simulink model "simulaciones_controlador"  (R2021a)
settings: Solver=VariableStepAuto  StartTime=0.0  StopTime=10.0  RelTol=1e-3
libraries: cstblocks x2
settings Model: Creator=camid  LastModifiedBy=camid

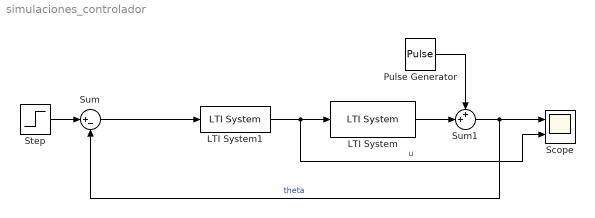
== system simulaciones_controlador ==
  LTI System : cstblocks/LTI System  sys=Planta  IC=[]
  LTI System1 : cstblocks/LTI System  sys=C  IC=[]
  Pulse Generator : DiscretePulseGenerator  PulseType=Time based  Amplitude=10  Period=30  PulseWidth=0.1  PhaseDelay=2
  Scope : Scope  NumInputPorts=2
  Step : Step  After=0  SampleTime=0
  Sum : Sum  Inputs=|+-
  Sum1 : Sum  Inputs=++|
  wires:
  Step/1 -> Sum/1
  Sum/1 -> LTI System1/1
  LTI System1/1 -> Scope/2, LTI System/1  "u"
  LTI System/1 -> Sum1/2
  Sum1/1 -> Sum/2, Scope/1  "theta"
  Pulse Generator/1 -> Sum1/1
